simulink model "test_compliance"  (R2023a)
settings: Solver=VariableStepAuto  StartTime=0.0  StopTime=10  RelTol=1e-3
undefined symbols (not defined in the file): dqi, K, KD, KP, qi, robot, xd, xr
settings Model: Creator=franc  LastModifiedBy=franc

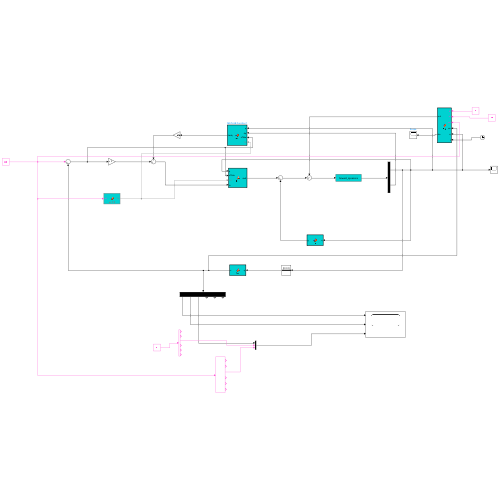
[thumbnail: Simulink's stored preview of the top-level diagram]
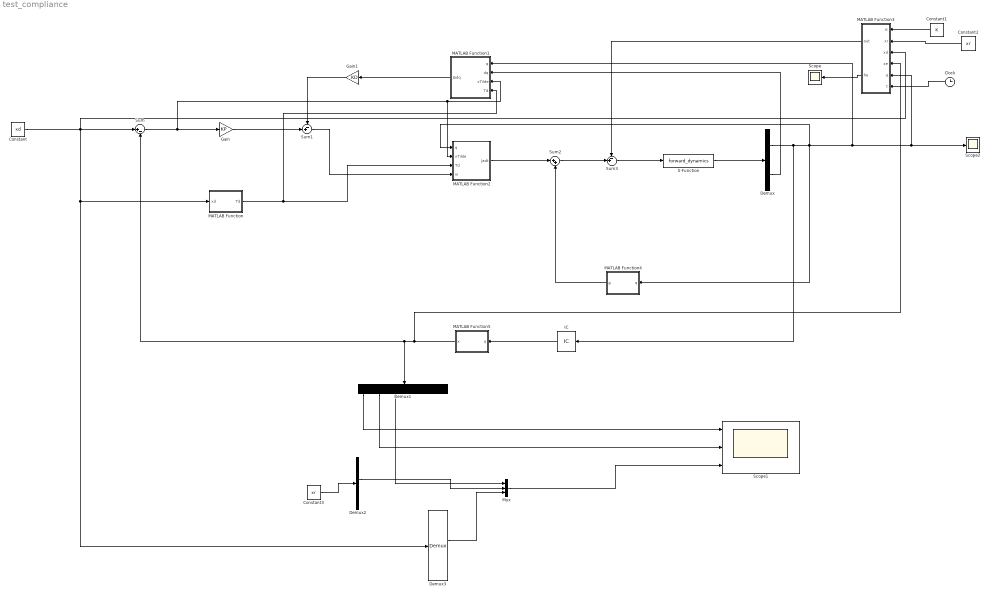
== system test_compliance ==
  Clock : Clock
  Constant : Constant  Value=xd
  Constant1 : Constant  Value=K
  Constant2 : Constant  Value=xr
  Constant3 : Constant  Value=xr
  Demux : Demux  Outputs=2
  Demux1 : Demux  Outputs=6
  Demux2 : Demux  Outputs=6
  Demux3 : Demux  Outputs=6
  Gain : Gain  Gain=KP
  Gain1 : Gain  Gain=KD
  IC : InitialCondition  Value=[0 0 0]
  MATLAB Function : MATLAB Function  TreatAsAtomicUnit=on
  MATLAB Function1 : MATLAB Function  TreatAsAtomicUnit=on
  MATLAB Function2 : MATLAB Function  TreatAsAtomicUnit=on
  MATLAB Function3 : MATLAB Function  TreatAsAtomicUnit=on
  MATLAB Function4 : MATLAB Function  TreatAsAtomicUnit=on
  MATLAB Function5 : MATLAB Function  TreatAsAtomicUnit=on
  Mux : Mux  Inputs=3
  S-Function : S-Function  FunctionName=forward_dynamics  Parameters=robot,qi,dqi  SFunctionDeploymentMode=off  EnableBusSupport=off
  Scope : Scope
  Scope1 : Scope  NumInputPorts=3
  Scope2 : Scope
  Sum : Sum  Inputs=|+-
  Sum1 : Sum  Inputs=-+|
  Sum2 : Sum  Inputs=|++
  Sum3 : Sum  Inputs=-+|
  wires:
  MATLAB Function4/1(g) -> Sum2/2
  Demux/1 -> IC/1, MATLAB Function1/1(q), Scope2/1, MATLAB Function3/5(q), MATLAB Function4/1(q), MATLAB Function2/1(q)
  Sum3/1 -> S-Function/1
  Sum2/1 -> Sum3/2
  MATLAB Function3/1(out) -> Sum3/1
  S-Function/1 -> Demux/1
  MATLAB Function2/1(Jadt) -> Sum2/1
  Gain1/1 -> Sum1/1
  MATLAB Function1/1(Jadq) -> Gain1/1
  Gain/1 -> Sum1/2
  MATLAB Function5/1(x) -> MATLAB Function3/4(xe), Demux1/1, Sum/2
  Constant/1 -> Demux3/1, MATLAB Function/1(xd), MATLAB Function3/3(xd), Sum/1
  Sum/1 -> Gain/1, MATLAB Function1/3(xTilde), MATLAB Function2/2(xTilde)
  MATLAB Function/1(Td) -> MATLAB Function2/3(Td), MATLAB Function1/4(Td)
  Sum1/1 -> MATLAB Function2/4(in)
  Demux/2 -> MATLAB Function1/2(dq)
  Constant1/1 -> MATLAB Function3/1(K)
  Constant2/1 -> MATLAB Function3/2(xr)
  MATLAB Function3/2(he) -> Scope/1
  IC/1 -> MATLAB Function5/1(q)
  Demux1/3 -> Mux/1
  Mux/1 -> Scope1/3
  Demux1/2 -> Scope1/2
  Demux1/1 -> Scope1/1
  Demux2/3 -> Mux/2
  Constant3/1 -> Demux2/1
  Demux3/3 -> Mux/3
  Clock/1 -> MATLAB Function3/6(t)

== matlab function test_compliance/MATLAB Function1 ==
  data: q input; Jadq output; dq input; xTilde input; Td input
function Jadq = fcn(q, dq,xTilde, Td)

Jadq = new_getJad(q,xTilde,Td)*dq;

== matlab function test_compliance/MATLAB Function ==
  data: xd input; Td output
function Td = getTd(xd)

%xd(4:6) are the phi angle
Rd = eul2rotm(xd(4:6)','ZYZ');
%xd(1:3) is the position 
t = xd(1:3);
Td = [Rd t
    zeros(1,3) 1];

== matlab function test_compliance/MATLAB Function2 ==
  data: q input; Jadt output; xTilde input; Td input; in input
function Jadt = fcn(q, xTilde, Td, in)

Jadt =new_getJad(q,xTilde,Td)'*in;

end

== matlab function test_compliance/MATLAB Function3 ==
  data: K input; out output; xr input; xd input; xe input; q input; he output; t input
function [out, he]= he(K, xr, xd, xe, q,t)
%consider the interaction only in z direction
q1 = q(1);
q2 = q(2);
q3 = q(3);
d0 = 0.15;
d1 = 0.4;
d2 = 0.3;
d3 = 0.24;

% if the end effector touch the environment 
he = zeros(6,1);

if xe(3) > xr(3)
    %The interaction force between the end-effector and the environment is
    if t == 0
        xe(3)
        xr(3)
        disp('HERE')
    end
    dxrd = xd-xr;
    dxed = xd-xe;
    dxre = dxrd-dxed;
    he = K*dxre;
end

Jtransp =[-sin(q1)*(d1 - d3*sin(q3)), cos(q1)*(d1 - d3*sin(q3)),           0, 1, 0, 0;
                         0,                         0,           1, 0, 0, 0;
       -d3*cos(q1)*cos(q3),       -d3*cos(q3)*sin(q1), -d3*sin(q3), 0, 0, 1];
 
%If there is interaction with the environment (hde != 0) the equilibrium will be at the pose
%Jtransp(q)* hde
out = Jtransp*he;

== matlab function test_compliance/MATLAB Function4 ==
  data: q input; g output
function g = G(q)

g = new_getG(q);

== matlab function test_compliance/MATLAB Function5 ==
  data: q input; x output
function x = fcn(q)

x = new_getK(q);
